simulink library "INT_Rail_MonMeUn"  (R2016b)
settings: Solver=VariableStepAuto  StartTime=0.0  StopTime=10.0  RelTol=1e-3
settings Model: Creator=liutao  LastModifiedBy=liutao

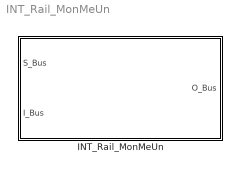
== system INT_Rail_MonMeUn ==
  INT_Rail_MonMeUn : Subsystem

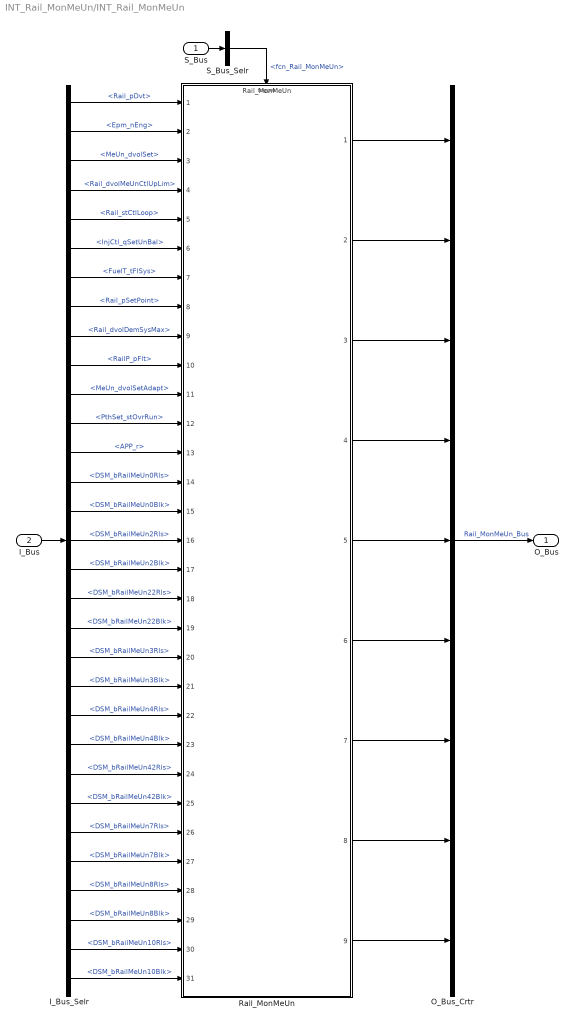
== system INT_Rail_MonMeUn/INT_Rail_MonMeUn ==
  S_Bus : Inport
  I_Bus : Inport  Port=2
  I_Bus_Selr : BusSelector  OutputSignals=Rail_pDvt,Epm_nEng,MeUn_dvolSet,Rail_dvolMeUnCtlUpLim,Rail_stCtlLoop,InjCtl_qSetUnBal,FuelT_tFlSys,Rail_pSetPoint,Rail_dvolDemSysMax,RailP_pFlt,MeUn_dvolSetAdapt,PthSet_stOvrRun,APP_r,DSM_bRailMeUn0Rls,DSM_bRailMeUn0Blk,DSM_bRailMeUn2Rls,DSM_bRailMeUn2Blk,DSM_bRailMeUn22Rls,DSM_bRailMeUn22Blk,DSM_bRailMeUn3Rls,DSM_bRailMeUn3Blk,DSM_bRailMeUn4Rls,DSM_bRailMeUn4Blk,DSM_bRailMeUn42Rls,DSM_bRailMeUn42Blk,DSM_bRailMeUn7Rls,DSM_bRailMeUn7Blk,DSM_bRailMeUn8Rls,DSM_bRailMeUn8Blk,DSM_bRailMeUn10Rls,DSM_bRailMeUn10Blk
  O_Bus_Crtr : BusCreator  Inputs=9
  Rail_MonMeUn : ModelReference  ModelNameDialog=Rail_MonMeUn  SimulationMode=Normal  ModelReferenceVersion=1.32  TriggerPortName=function  TriggerPortTriggerType=function-call  TriggerPortStatesWhenEnabling=held
  S_Bus_Selr : BusSelector  OutputSignals=fcn_Rail_MonMeUn
  O_Bus : Outport
  wires:
  S_Bus_Selr/1 -> Rail_MonMeUn/Trigger  "<fcn_Rail_MonMeUn>"
  S_Bus/1 -> S_Bus_Selr/1
  I_Bus/1 -> I_Bus_Selr/1
  I_Bus_Selr/1 -> Rail_MonMeUn/1  "<Rail_pDvt>"
  I_Bus_Selr/2 -> Rail_MonMeUn/2  "<Epm_nEng>"
  I_Bus_Selr/3 -> Rail_MonMeUn/3  "<MeUn_dvolSet>"
  I_Bus_Selr/4 -> Rail_MonMeUn/4  "<Rail_dvolMeUnCtlUpLim>"
  I_Bus_Selr/5 -> Rail_MonMeUn/5  "<Rail_stCtlLoop>"
  I_Bus_Selr/6 -> Rail_MonMeUn/6  "<InjCtl_qSetUnBal>"
  I_Bus_Selr/7 -> Rail_MonMeUn/7  "<FuelT_tFlSys>"
  I_Bus_Selr/8 -> Rail_MonMeUn/8  "<Rail_pSetPoint>"
  I_Bus_Selr/9 -> Rail_MonMeUn/9  "<Rail_dvolDemSysMax>"
  I_Bus_Selr/10 -> Rail_MonMeUn/10  "<RailP_pFlt>"
  I_Bus_Selr/11 -> Rail_MonMeUn/11  "<MeUn_dvolSetAdapt>"
  I_Bus_Selr/12 -> Rail_MonMeUn/12  "<PthSet_stOvrRun>"
  I_Bus_Selr/13 -> Rail_MonMeUn/13  "<APP_r>"
  I_Bus_Selr/14 -> Rail_MonMeUn/14  "<DSM_bRailMeUn0Rls>"
  I_Bus_Selr/15 -> Rail_MonMeUn/15  "<DSM_bRailMeUn0Blk>"
  I_Bus_Selr/16 -> Rail_MonMeUn/16  "<DSM_bRailMeUn2Rls>"
  I_Bus_Selr/17 -> Rail_MonMeUn/17  "<DSM_bRailMeUn2Blk>"
  I_Bus_Selr/18 -> Rail_MonMeUn/18  "<DSM_bRailMeUn22Rls>"
  I_Bus_Selr/19 -> Rail_MonMeUn/19  "<DSM_bRailMeUn22Blk>"
  I_Bus_Selr/20 -> Rail_MonMeUn/20  "<DSM_bRailMeUn3Rls>"
  I_Bus_Selr/21 -> Rail_MonMeUn/21  "<DSM_bRailMeUn3Blk>"
  I_Bus_Selr/22 -> Rail_MonMeUn/22  "<DSM_bRailMeUn4Rls>"
  I_Bus_Selr/23 -> Rail_MonMeUn/23  "<DSM_bRailMeUn4Blk>"
  I_Bus_Selr/24 -> Rail_MonMeUn/24  "<DSM_bRailMeUn42Rls>"
  I_Bus_Selr/25 -> Rail_MonMeUn/25  "<DSM_bRailMeUn42Blk>"
  I_Bus_Selr/26 -> Rail_MonMeUn/26  "<DSM_bRailMeUn7Rls>"
  I_Bus_Selr/27 -> Rail_MonMeUn/27  "<DSM_bRailMeUn7Blk>"
  I_Bus_Selr/28 -> Rail_MonMeUn/28  "<DSM_bRailMeUn8Rls>"
  I_Bus_Selr/29 -> Rail_MonMeUn/29  "<DSM_bRailMeUn8Blk>"
  I_Bus_Selr/30 -> Rail_MonMeUn/30  "<DSM_bRailMeUn10Rls>"
  I_Bus_Selr/31 -> Rail_MonMeUn/31  "<DSM_bRailMeUn10Blk>"
  O_Bus_Crtr/1 -> O_Bus/1  "Rail_MonMeUn_Bus"
  Rail_MonMeUn/1 -> O_Bus_Crtr/1
  Rail_MonMeUn/2 -> O_Bus_Crtr/2
  Rail_MonMeUn/3 -> O_Bus_Crtr/3
  Rail_MonMeUn/4 -> O_Bus_Crtr/4
  Rail_MonMeUn/5 -> O_Bus_Crtr/5
  Rail_MonMeUn/6 -> O_Bus_Crtr/6
  Rail_MonMeUn/7 -> O_Bus_Crtr/7
  Rail_MonMeUn/8 -> O_Bus_Crtr/8
  Rail_MonMeUn/9 -> O_Bus_Crtr/9
